simulink model "fuzzy_system"  (R2018b)
settings: Solver=VariableStepAuto  StartTime=0.0  StopTime=10  RelTol=1e-3
undefined symbols (not defined in the file or in its folder): tanks_level_system
libraries: simulink x1
settings Model: Creator=fredericovaz  LastModifiedBy=fred

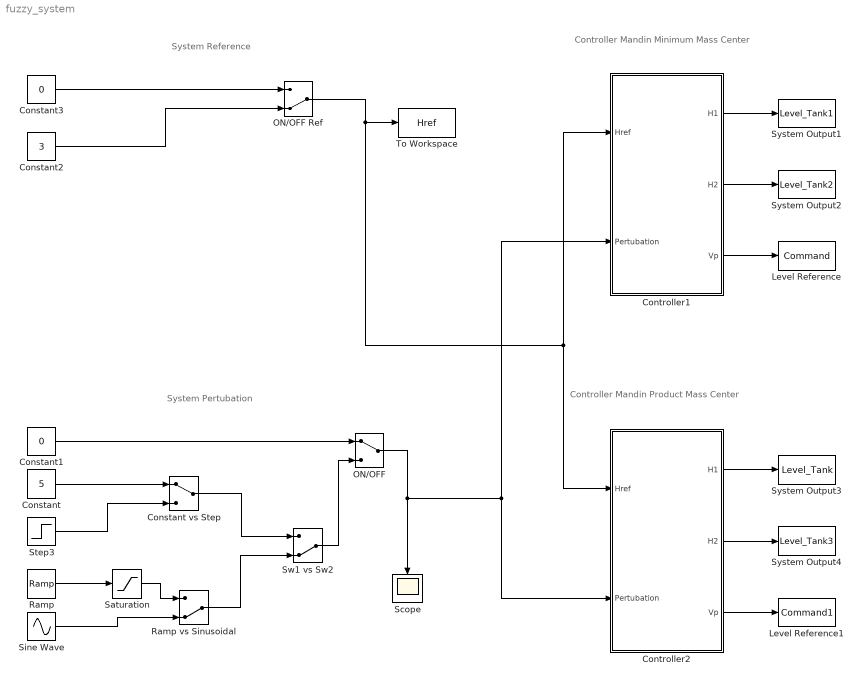
== system fuzzy_system ==
  note: Controller Mandin Minimum Mass Center
  note: Controller Mandin Product Mass Center
  note: System Pertubation
  note: System Reference
  Constant : Constant  Value=5
  Constant vs Step : ManualSwitch
  Constant1 : Constant  Value=0
  Constant2 : Constant  Value=3
  Constant3 : Constant  Value=0
  Controller1 : Subsystem
  Controller2 : Subsystem
  Level Reference : ToWorkspace  VariableName=Command  SaveFormat=Timeseries  SampleTime=-1
  Level Reference1 : ToWorkspace  VariableName=Command1  SaveFormat=Timeseries  SampleTime=-1
  ON/OFF : ManualSwitch
  ON/OFF Ref : ManualSwitch  CurrentSetting=0
  Ramp : simulink/Sources/Ramp  slope=2  start=60  InitialOutput=0
  Ramp vs Sinusoidal : ManualSwitch  CurrentSetting=0
  Saturation : Saturate  UpperLimit=5  LowerLimit=0
  Scope : Scope
  Sine Wave : Sin  Amplitude=5  Frequency=20  SampleTime=0
  Step3 : Step  Time=60  After=5  SampleTime=0
  Sw1 vs Sw2 : ManualSwitch  CurrentSetting=0
  System Output1 : ToWorkspace  VariableName=Level_Tank1  SaveFormat=Timeseries  SampleTime=-1
  System Output2 : ToWorkspace  VariableName=Level_Tank2  SaveFormat=Timeseries  SampleTime=-1
  System Output3 : ToWorkspace  VariableName=Level_Tank  SaveFormat=Timeseries  SampleTime=-1
  System Output4 : ToWorkspace  VariableName=Level_Tank3  SaveFormat=Timeseries  SampleTime=-1
  To Workspace : ToWorkspace  VariableName=Href  SaveFormat=Timeseries  SampleTime=-1
  wires:
  ON/OFF Ref/1 -> Controller2/1(Href), Controller1/1(Href), To Workspace/1
  Controller1/2(H2) -> System Output2/1
  Controller1/3(Vp) -> Level Reference/1
  Controller1/1(H1) -> System Output1/1
  Controller2/3(Vp) -> Level Reference1/1
  Controller2/1(H1) -> System Output3/1
  Controller2/2(H2) -> System Output4/1
  ON/OFF/1 -> Scope/1, Controller1/2(Pertubation), Controller2/2(Pertubation)
  Saturation/1 -> Ramp vs Sinusoidal/1
  Constant/1 -> Constant vs Step/1
  Ramp vs Sinusoidal/1 -> Sw1 vs Sw2/2
  Constant vs Step/1 -> Sw1 vs Sw2/1
  Sine Wave/1 -> Ramp vs Sinusoidal/2
  Step3/1 -> Constant vs Step/2
  Ramp/1 -> Saturation/1
  Constant1/1 -> ON/OFF/1
  Sw1 vs Sw2/1 -> ON/OFF/2
  Constant3/1 -> ON/OFF Ref/1
  Constant2/1 -> ON/OFF Ref/2

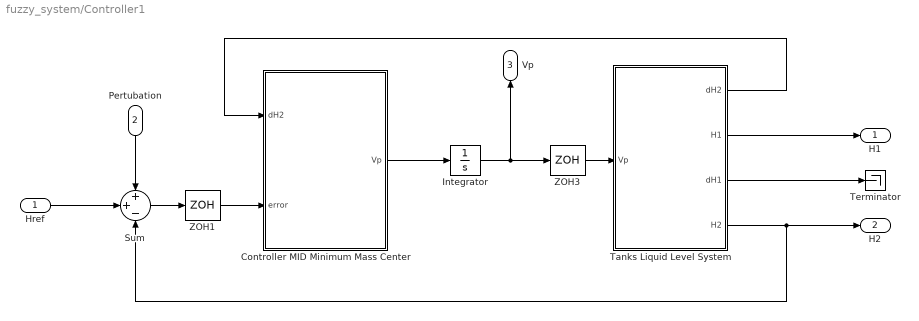
== system fuzzy_system/Controller1 ==
  Href : Inport
  Pertubation : Inport  Port=2
  Controller MID Minimum Mass Center : MATLAB Function  TreatAsAtomicUnit=on
  Integrator : Integrator
  Sum : Sum  Inputs=++-
  Tanks Liquid Level System : Subsystem
  Terminator : Terminator
  ZOH1 : ZeroOrderHold  SampleTime=1e-3
  ZOH3 : ZeroOrderHold  SampleTime=1e-3
  H1 : Outport
  H2 : Outport  Port=2
  Vp : Outport  Port=3
  wires:
  Tanks Liquid Level System/4(H2) -> H2/1, Sum/3
  Tanks Liquid Level System/1(dH2) -> Controller MID Minimum Mass Center/1(dH2)
  Tanks Liquid Level System/2(H1) -> H1/1
  ZOH3/1 -> Tanks Liquid Level System/1(Vp)
  Integrator/1 -> Vp/1, ZOH3/1
  Controller MID Minimum Mass Center/1(Vp) -> Integrator/1
  Tanks Liquid Level System/3("dH1 ") -> Terminator/1
  Sum/1 -> ZOH1/1
  Pertubation/1 -> Sum/1
  Href/1 -> Sum/2
  ZOH1/1 -> Controller MID Minimum Mass Center/2(error)

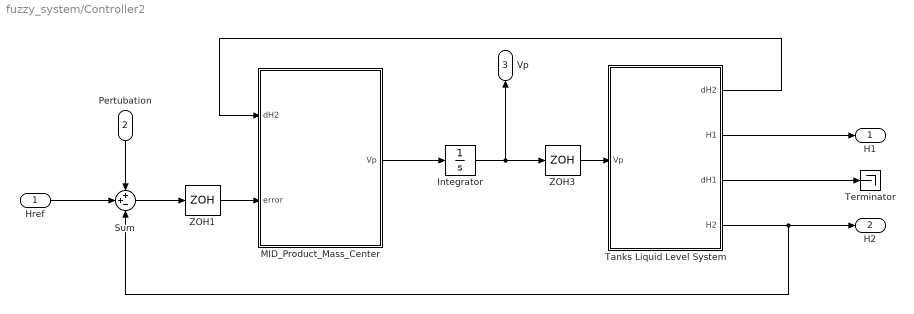
== system fuzzy_system/Controller2 ==
  Href : Inport
  Pertubation : Inport  Port=2
  Integrator : Integrator
  MID_Product_Mass_Center : MATLAB Function  TreatAsAtomicUnit=on
  Sum : Sum  Inputs=++-
  Tanks Liquid Level System : Subsystem
  Terminator : Terminator
  ZOH1 : ZeroOrderHold  SampleTime=1e-3
  ZOH3 : ZeroOrderHold  SampleTime=1e-3
  H1 : Outport
  H2 : Outport  Port=2
  Vp : Outport  Port=3
  wires:
  Tanks Liquid Level System/4(H2) -> H2/1, Sum/3
  Tanks Liquid Level System/1(dH2) -> MID_Product_Mass_Center/1(dH2)
  Tanks Liquid Level System/2(H1) -> H1/1
  ZOH3/1 -> Tanks Liquid Level System/1(Vp)
  ZOH1/1 -> MID_Product_Mass_Center/2(error)
  Sum/1 -> ZOH1/1
  Integrator/1 -> Vp/1, ZOH3/1
  MID_Product_Mass_Center/1(Vp) -> Integrator/1
  Tanks Liquid Level System/3("dH1 ") -> Terminator/1
  Href/1 -> Sum/2
  Pertubation/1 -> Sum/1

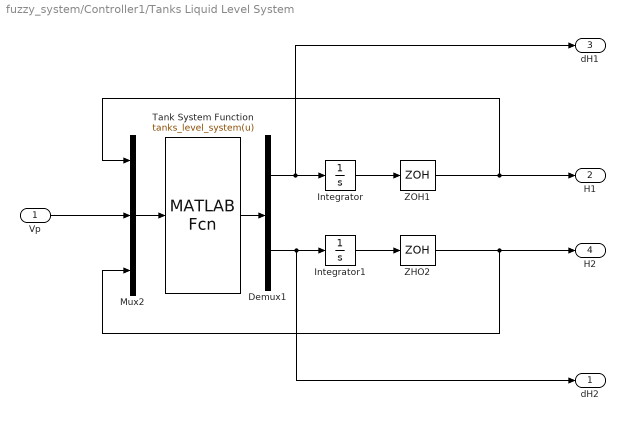
== system fuzzy_system/Controller1/Tanks Liquid Level System ==
  Vp : Inport
  Demux1 : Demux  Outputs=2
  Integrator : Integrator
  Integrator1 : Integrator
  Mux2 : Mux  Inputs=3
  Tank System Function : MATLABFcn  MATLABFcn=tanks_level_system(u)  OutputDimensions=2
  ZHO2 : ZeroOrderHold  SampleTime=1e-3
  ZOH1 : ZeroOrderHold  SampleTime=1e-3
  dH2 : Outport
  H1 : Outport  Port=2
  "dH1 " : Outport  Port=3
  H2 : Outport  Port=4
  wires:
  Demux1/2 -> Integrator1/1, dH2/1
  Integrator1/1 -> ZHO2/1
  Vp/1 -> Mux2/2
  ZHO2/1 -> H2/1, Mux2/3
  Integrator/1 -> ZOH1/1
  Tank System Function/1 -> Demux1/1
  ZOH1/1 -> H1/1, Mux2/1
  Demux1/1 -> Integrator/1, "dH1 "/1
  Mux2/1 -> Tank System Function/1

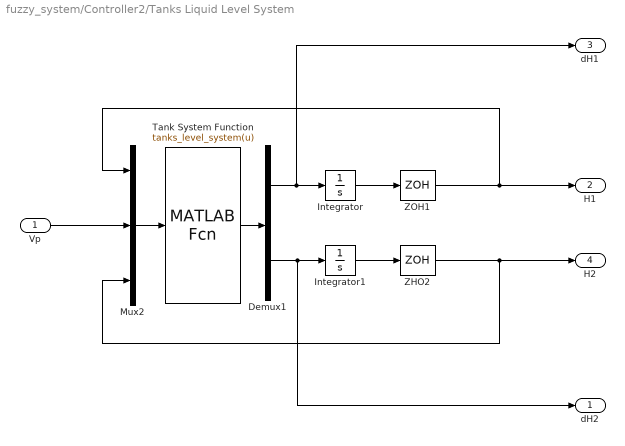
== system fuzzy_system/Controller2/Tanks Liquid Level System ==
  Vp : Inport
  Demux1 : Demux  Outputs=2
  Integrator : Integrator
  Integrator1 : Integrator
  Mux2 : Mux  Inputs=3
  Tank System Function : MATLABFcn  MATLABFcn=tanks_level_system(u)  OutputDimensions=2
  ZHO2 : ZeroOrderHold  SampleTime=1e-3
  ZOH1 : ZeroOrderHold  SampleTime=1e-3
  dH2 : Outport
  H1 : Outport  Port=2
  "dH1 " : Outport  Port=3
  H2 : Outport  Port=4
  wires:
  Demux1/2 -> Integrator1/1, dH2/1
  Integrator1/1 -> ZHO2/1
  Vp/1 -> Mux2/2
  ZHO2/1 -> H2/1, Mux2/3
  Integrator/1 -> ZOH1/1
  Tank System Function/1 -> Demux1/1
  ZOH1/1 -> H1/1, Mux2/1
  Demux1/1 -> Integrator/1, "dH1 "/1
  Mux2/1 -> Tank System Function/1

== matlab function fuzzy_system/Controller2/MID_Product_Mass_Center ==
  data: dH2 input; error input; Vp output

%%

function Vp  = fcn(dH2, error)


Vp = error;


end

== matlab function fuzzy_system/Controller1/Controller MID Minimum Mass Center ==
  data: dH2 input; Vp output; error input

function Vp  = fcn(dH2, error) % dH2, Href, H2
%% Controller Minimum Mass Center Function
%   - Triangular Diffuser
%   - Motor de Inferência de Mínimo
%   - Desdifusor por Centro de Massa

%--------------------------------------------------------------------------
% Init
%--------------------------------------------------------------------------

dH2_ = zeros(5);
error_ = zeros(5);


%--------------------------------------------------------------------------
% Diffusers and Trust Values
%--------------------------------------------------------------------------

% Reference between Tank2 Level (H2) 
error_(1) = error_MH(error);                   % Much Higher
error_(2) = error_H(error);                    % Higher 
error_(3) = error_N(error);                    % Near
error_(4) = error_L(error);                    % Lower
error_(5) = error_ML(error);                   % Much Lower


% Tank2 Level Variation: dH2 
dH2_(1) = dH2_DF(dH2);                         % Down Fast
dH2_(2) = dH2_D(dH2);                          % Down
dH2_(3) = dH2_S(dH2);                          % Slow
dH2_(4) = dH2_U(dH2);                          % Up
dH2_(5) = dH2_UF(dH2);                         % Up Fast



 

% 
% [] = MID_Mamdani_min(Vp_dH2, Vp_error);
% 
% 






Vp = error;

end






% % Error between -100 and 100
% error = ((Href - H2)/100)*100;
% 
% % Normalized dH2
% dH2_norm = dH2/abs(error);


%--------------------------------------------------------------------------
% Diffusers
%--------------------------------------------------------------------------

% Tank2 Level Variation: dH2 

% [ dif_MU,dif_U,dif_A,dif_D,dif_MD ] = fuzzy1();
% 
% % More UP
% % UP
% % Slow
% % Down
% % More Down
% 
% % Voltage Motor Variation: dVp
% [ DM, dif_D, M, I, IM] = fuzzy2();


%--------------------------------------------------------------------------
% Trust Values
%--------------------------------------------------------------------------
